simulink model "darko_test_integrateur"  (R2021b)
settings: Solver=VariableStepAuto  StartTime=0.0  StopTime=30  RelTol=1e-3
values from neighbouring files (symbols this model uses):
  drone = generateDarko()    [main_linearisation.m]
  initial_state = [p_initial; v_initial; q_initial; omega_initial]    [main_linearisation.m]
  K_complet = [K(:,1:6), zeros(4,1), K(:,7:12)]    [main_linearisation.m]
  S_complet = [S(1:6,1:6), zeros(6,1), S(1:6,7:12); zeros(1,13); S(7:12,1:6), zeros(6,1), S(7:12,7:12)]    [main_linearisation.m]
  u_eq = drone.G*drone.MASS/(2*drone.Fb(1,1)) * [1;1;0;0]    [main_linearisation.m]
  x_eq = [[0; 0; 0]; [0; 0; 0]; eul2quat([yaw, pitch, roll])'; [0; 0; 0]]    [main_linearisation.m]
libraries: simulink_extras x3, sharedtransform x1
settings Model: Creator=florian  LastModifiedBy=florian
settings SolverCC: AlgebraicLoopSolver=TrustRegion
settings DebuggingCC: SFMachineParentedDataDiag=warning

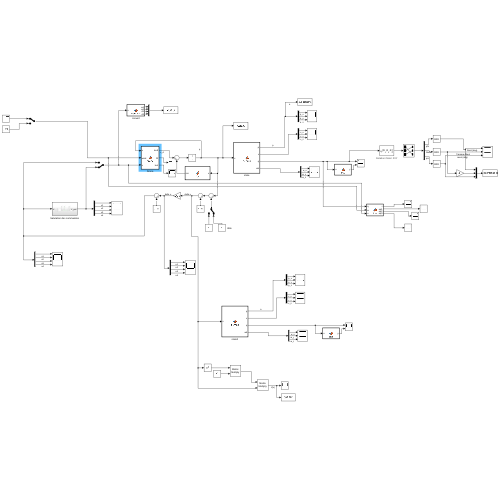
[thumbnail: Simulink's stored preview of the top-level diagram]
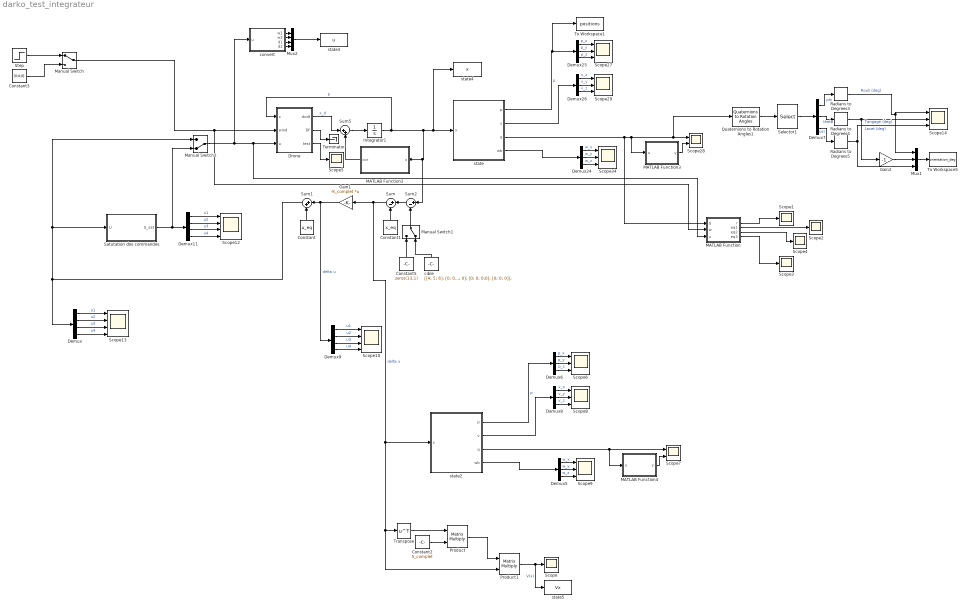
== system darko_test_integrateur ==
  Constant : Constant  Value=u_eq
  Constant1 : Constant  Value=x_eq
  Constant2 : Constant  Value=S_complet
  Constant3 : Constant  Value=[0;0;0]
  Constant5 : Constant  Value=zeros(13,1)
  Demux : Demux
  Demux11 : Demux
  Demux{5..8,24..26} (7 alike) : Demux  Outputs=3
  Demux9 : Demux
  Drone : MATLAB Function  TreatAsAtomicUnit=on
  Gain1 : Gain  Gain=-K_complet  Multiplication=Matrix(K*u) (u vector)
  Gain2 : Gain  Gain=-1
  Integrator1 : Integrator  InitialCondition=initial_state
  MATLAB Function : MATLAB Function  TreatAsAtomicUnit=on
  MATLAB Function2 : MATLAB Function  TreatAsAtomicUnit=on
  MATLAB Function3 : MATLAB Function  TreatAsAtomicUnit=on
  MATLAB Function4 : MATLAB Function  TreatAsAtomicUnit=on
  Manual Switch : ManualSwitch
  Manual Switch1 : ManualSwitch  CurrentSetting=0
  Manual Switch2 : ManualSwitch  CurrentSetting=0
  Mux1 : Mux  Inputs=3
  Mux2 : Mux
  Product : Product  Multiplication=Matrix(*)
  Product1 : Product  Multiplication=Matrix(*)
  Quaternions to Rotation Angles1 : sharedtransform/Quaternions to Rotation Angles  rotationOrder=ZXY  aMode=aMode
      settings: SourceProductBaseCode=AE,PW,DR,MT,UV,VE
  Radians to Degrees3 : simulink_extras/Transformations/Radians to Degrees
  Radians to Degrees4 : simulink_extras/Transformations/Radians to Degrees
  Radians to Degrees5 : simulink_extras/Transformations/Radians to Degrees
  Satutation des commandes : Subsystem
  Scope{,1..5} (6 alike) : Scope
  Scope10 : Scope  NumInputPorts=4
  Scope12 : Scope  NumInputPorts=4
  Scope13 : Scope  NumInputPorts=4
  Scope{6,8..9,14,27,29,34} (7 alike) : Scope  NumInputPorts=3
  Scope28 : Scope  NumInputPorts=2
  Scope7 : Scope  NumInputPorts=2
  Selector1 : Selector  InputPortWidth=3  IndexOptions=Index vector (dialog)  Indices=[2 3 1]  OutputSizes=1
  Step : Step  Time=10  Before=[0;0;0]  After=[0;0;-10]  SampleTime=0
  Sum : Sum  Inputs=|+-
  Sum1 : Sum  Inputs=|++
  Sum2 : Sum  Inputs=|+-
  Sum5 : Sum  Inputs=|++
  Terminator : Terminator
  To Workspace1 : ToWorkspace  VariableName=positions  SampleTime=-1
  To Workspace5 : ToWorkspace  VariableName=orientation_deg  SampleTime=-1
  Transpose : Math  Operator=transpose  SaturateOnIntegerOverflow=on
  cible : Constant  Value=[[4; 5; 6]; [0; 0; 0]; [0; 0; 0;0]; [0; 0; 0]];
  convert : MATLAB Function  TreatAsAtomicUnit=on
  state : MATLAB Function  TreatAsAtomicUnit=on
  state2 : MATLAB Function  TreatAsAtomicUnit=on
  state3 : ToWorkspace  VariableName=u  SampleTime=-1
  state4 : ToWorkspace  VariableName=x  SampleTime=-1
  state5 : ToWorkspace  VariableName=Vx  SampleTime=-1
  wires:
  Sum5/1 -> Integrator1/1
  MATLAB Function2/1(cor) -> Sum5/2
  Drone/1(dxdt) -> Sum5/1  "x_d"
  Integrator1/1 -> Drone/1(x), state4/1, state/1(x), Sum2/1, MATLAB Function2/1(x)  "p"
  Demux25/3 -> Scope27/3  "p_z"
  Demux26/2 -> Scope29/2  "v_y"
  Demux24/1 -> Scope34/1  "w_x"
  MATLAB Function3/1(y) -> Scope28/2
  state/3(q) -> MATLAB Function/1(q), MATLAB Function3/1(u), Quaternions to Rotation Angles1/1, Scope28/1
  Demux25/1 -> Scope27/1  "p_x"
  state/4(wb) -> Demux24/1
  Demux24/2 -> Scope34/2  "w_y"
  Demux24/3 -> Scope34/3  "w_z"
  state/2(v) -> Demux26/1
  Demux25/2 -> Scope27/2  "p_y"
  Demux26/3 -> Scope29/3  "v_z"
  Demux26/1 -> Scope29/1  "v_x"
  Gain1/1 -> Demux9/1, Sum1/1  "delta u"
  Constant/1 -> Sum1/2
  Constant1/1 -> Sum/2
  Demux6/3 -> Scope6/3  "p_z"
  Demux8/2 -> Scope8/2  "v_y"
  state2/3(q) -> MATLAB Function4/1(u), Scope7/1
  state2/4(wb) -> Demux5/1
  MATLAB Function4/1(y) -> Scope7/2
  Demux5/2 -> Scope9/2  "w_y"
  Demux8/3 -> Scope8/3  "v_z"
  Demux6/1 -> Scope6/1  "p_x"
  Demux5/1 -> Scope9/1  "w_x"
  Demux8/1 -> Scope8/1  "v_x"
  state2/1(p) -> Demux6/1  "p"
  Demux6/2 -> Scope6/2  "p_y"
  Demux5/3 -> Scope9/3  "w_z"
  state2/2(v) -> Demux8/1
  Demux9/3 -> Scope10/3  "u3"
  Demux9/4 -> Scope10/4  "u4"
  Demux9/1 -> Scope10/1  "u1"
  Demux9/2 -> Scope10/2  "u2"
  Product1/1 -> state5/1, Scope/1  "V(x)"
  Transpose/1 -> Product/1
  Constant2/1 -> Product/2
  Product/1 -> Product1/1
  Manual Switch/1 -> MATLAB Function/2(w), Drone/2(wind)
  Step/1 -> Manual Switch/1
  Constant3/1 -> Manual Switch/2
  cible/1 -> Manual Switch1/2
  Manual Switch1/1 -> Sum2/2
  Constant5/1 -> Manual Switch1/1
  Sum2/1 -> Sum/1
  Demux/1 -> Scope13/1  "u1"
  Demux11/2 -> Scope12/2  "u2"
  Demux11/4 -> Scope12/4  "u4"
  Demux/2 -> Scope13/2  "u2"
  Demux/4 -> Scope13/4  "u4"
  Demux11/1 -> Scope12/1  "u1"
  Demux/3 -> Scope13/3  "u3"
  Sum1/1 -> Satutation des commandes/1(U), Manual Switch2/1, Demux/1
  Satutation des commandes/1(U_sat) -> Manual Switch2/2, Demux11/1
  Demux11/3 -> Scope12/3  "u3"
  Manual Switch2/1 -> convert/1(u), MATLAB Function/3(u), Drone/3(u)
  Sum/1 -> Product1/2, Transpose/1, state2/1(x), Gain1/1  "delta x"
  Demux7/2 -> Radians to Degrees4/1  "theta"
  Radians to Degrees4/1 -> Gain2/1, Scope14/2  "Tangage (deg)"
  Gain2/1 -> Mux1/2
  Mux1/1 -> To Workspace5/1
  Radians to Degrees5/1 -> Mux1/3, Scope14/3  "Lacet (deg)"
  Quaternions to Rotation Angles1/1 -> Selector1/1
  Demux7/3 -> Radians to Degrees5/1  "psi"
  Selector1/1 -> Demux7/1
  Demux7/1 -> Radians to Degrees3/1  "phi"
  Radians to Degrees3/1 -> Mux1/1, Scope14/1  "Rouli (deg)"
  state/1(p) -> To Workspace1/1, Demux25/1  "p"
  convert/2(w2) -> Mux2/2
  convert/4(d2) -> Mux2/4
  convert/3(d1) -> Mux2/3
  Mux2/1 -> state3/1
  convert/1(w1) -> Mux2/1
  MATLAB Function/1(r) -> Scope1/1
  MATLAB Function/2(eq1) -> Scope2/1
  MATLAB Function/4(eq3) -> Scope3/1
  MATLAB Function/3(eq2) -> Scope4/1
  Drone/2(Df) -> Terminator/1
  Drone/3(test) -> Scope5/1

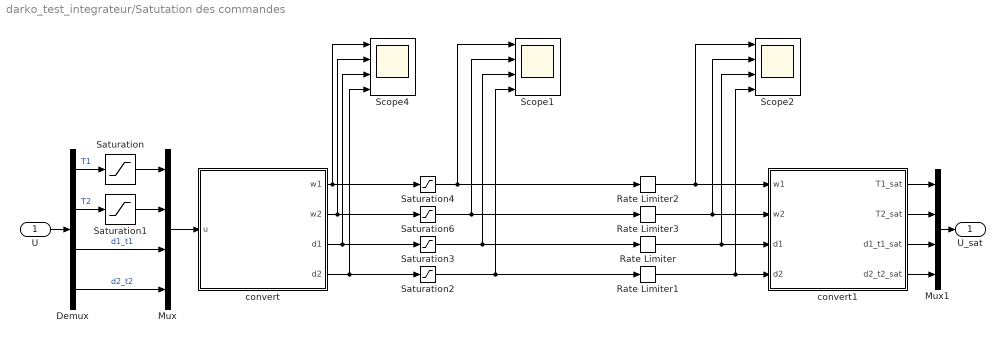
== system darko_test_integrateur/Satutation des commandes ==
  U : Inport
  Demux : Demux
  Mux : Mux
  Mux1 : Mux
  Rate Limiter : RateLimiter  RisingSlewLimit=drone.ELEVON_RATE_CHANGE  FallingSlewLimit=-drone.ELEVON_RATE_CHANGE  SampleTimeMode=inherited
  Rate Limiter1 : RateLimiter  RisingSlewLimit=drone.ELEVON_RATE_CHANGE  FallingSlewLimit=-drone.ELEVON_RATE_CHANGE  SampleTimeMode=inherited
  Rate Limiter2 : RateLimiter  RisingSlewLimit=drone.MOTOR_RATE_CHANGE  FallingSlewLimit=-drone.MOTOR_RATE_CHANGE  SampleTimeMode=inherited
  Rate Limiter3 : RateLimiter  RisingSlewLimit=drone.MOTOR_RATE_CHANGE  FallingSlewLimit=-drone.MOTOR_RATE_CHANGE  SampleTimeMode=inherited
  Saturation : Saturate  UpperLimit=100  LowerLimit=0.001
  Saturation1 : Saturate  UpperLimit=100  LowerLimit=0.001
  Saturation2 : Saturate  UpperLimit=30*(pi/180)  LowerLimit=-30*(pi/180)
  Saturation3 : Saturate  UpperLimit=30*(pi/180)  LowerLimit=-30*(pi/180)
  Saturation4 : Saturate  UpperLimit=1000  LowerLimit=200
  Saturation6 : Saturate  UpperLimit=1000  LowerLimit=200
  Scope1 : Scope  NumInputPorts=4
  Scope2 : Scope  NumInputPorts=4
  Scope4 : Scope  NumInputPorts=4
  convert : MATLAB Function  TreatAsAtomicUnit=on
  convert1 : MATLAB Function  TreatAsAtomicUnit=on
  U_sat : Outport
  wires:
  U/1 -> Demux/1
  Demux/4 -> Mux/4  "d2_t2"
  Demux/1 -> Saturation/1  "T1"
  Demux/3 -> Mux/3  "d1_t1"
  Demux/2 -> Saturation1/1  "T2"
  Saturation/1 -> Mux/1
  Mux/1 -> convert/1(u)
  convert/1(w1) -> Saturation4/1, Scope4/1
  Saturation3/1 -> Rate Limiter/1, Scope1/3
  convert/2(w2) -> Scope4/2, Saturation6/1
  convert/3(d1) -> Scope4/3, Saturation3/1
  convert/4(d2) -> Saturation2/1, Scope4/4
  convert1/1(T1_sat) -> Mux1/1
  convert1/4(d2_t2_sat) -> Mux1/4
  Mux1/1 -> U_sat/1
  Saturation1/1 -> Mux/2
  convert1/2(T2_sat) -> Mux1/2
  convert1/3(d1_t1_sat) -> Mux1/3
  Saturation2/1 -> Rate Limiter1/1, Scope1/4
  Rate Limiter/1 -> Scope2/3, convert1/3(d1)
  Saturation6/1 -> Rate Limiter3/1, Scope1/2
  Saturation4/1 -> Rate Limiter2/1, Scope1/1
  Rate Limiter1/1 -> Scope2/4, convert1/4(d2)
  Rate Limiter2/1 -> Scope2/1, convert1/1(w1)
  Rate Limiter3/1 -> Scope2/2, convert1/2(w2)

== matlab function darko_test_integrateur/state ==
  data: x input; p output; v output; q output; wb output
function [p, v, q, wb] = demux(x)
%#codegen

p = x(1:3);
v = x(4:6);
q  = x(7:10);
wb = x(11:13);

== matlab function darko_test_integrateur/MATLAB Function ==
  data: q input; w input; u input; r output; drone parameter; eq1 output; eq2 output; eq3 output
function [r,eq1,eq2,eq3] = fcn(q,w,u,drone)
%#codegen
theta=2*asin(q(3));

rho = drone.RHO;
Swet   = drone.WET_SURFACE;
Sp = pi*drone.PROP_RADIUS^2;
Thetam = drone.ELEVON_MEFFICIENCY;
Thetaf = drone.ELEVON_FEFFICIENCY;
Cd0 = drone.PHI(1,1);
Cl0 = drone.PHI(3,3);
g = drone.G;
% vehicle mass
m = drone.MASS;


mu=(1-Thetaf(2)/Thetam(2))*(Swet*Cl0*rho)/(2*m*g);

r=mu*w(1)*sin(theta)-(mu*w(3)-1)*cos(theta);

wx_b = cos(theta)*w(1) + sin(theta)*w(3);
wz_b = cos(theta)*w(3) - sin(theta)*w(1);

eq1=rho*Thetam(2)*(u(3)/u(1))*wx_b + rho*wz_b + (1/Sp)*Thetam(2)*u(3);

eq2 = sin(theta)*m*g +2*(1-(Swet/4*Sp)*Cd0)*u(1) + (1/2)*rho*Swet*Cd0*(wx_b-Thetaf(2)*(u(1)/u(3))*wz_b);

eq3 = -cos(theta)*m*g +2*(-(Swet/4*Sp)*Cl0*Thetaf(2))*u(3) + (1/2)*rho*Swet*Cl0*(wz_b + Thetaf(2)*(u(1)/u(3))*wx_b);

== matlab function darko_test_integrateur/Drone ==
  data: x input; wind input; u input; dxdt output; drone parameter; Df output; test output
function [dxdt, Df, test]   = drone(x,wind, u, drone)

%% physical constants
% gravity
g = drone.G;
% vehicle mass
m = drone.MASS;
% vehicle inertia matrix
J = drone.INERTIA; % [3x3 real symmetric] in body axis

rho = drone.RHO;
Swet   = drone.WET_SURFACE;
Sp = pi*drone.PROP_RADIUS^2;
Thetam = drone.ELEVON_MEFFICIENCY;
Thetaf = drone.ELEVON_FEFFICIENCY;
Cd0 = drone.PHI(1,1);
Cl0 = drone.PHI(3,3);
dR = drone.CENTRAGE ;

af = drone.Fb(1,1);
bf = drone.Fb(3,3);

%% state demultiplexing
% p = x(1:3);
v = x(4:6);
q  = x(7:10);
wb = x(11:13);

Rq = q2dcm(q);

[Fp, Mp] = external_force_moment(x, u, wind, drone);

% position
dpdt = v;

Df = -(1/4)*rho*Swet*[-2*Cd0 0 Cd0*Thetaf(2)*((u(3)/u(1))+(u(4)/u(2))); 0 0 0; -Thetaf(2)*Cl0*((u(3)/u(1))+(u(4)/u(2))) 0 -2*Cl0];
test=norm(Rq*Df*Rq'*norm(wind)*wind)
% kinematics
dvdt =  -[0;0;g] + (1/m)*Rq*drone.Fb*u + (1/m)*Rq*Df*Rq'*norm(wind)*wind; 

%% quaternion derivative
eta = q(1);
eps = q(2:4);

dqdt = (1/2)*[-eps'; eta*eye(3) + skew_sym(eps)]*wb;

%% angular velocity derivative
Dm = -(1/4)*rho*Swet*[0 0 0; dR*Thetam(2)*Cl0*((u(3)/u(1))+(u(4)/u(2))) 0 -2*dR*Cl0; 0 0 0];
% kinematics
dwdt = inv(J)*(-cross(wb, J*wb) + (drone.Mb*u) + Dm*Rq'*norm(wind)*wind);


%% derivative multiplexing
dxdt = [dpdt; dvdt; dqdt; dwdt] ;

== matlab function darko_test_integrateur/MATLAB Function4 ==
  data: u input; y output
function y = fcn(u)
%#codegen

y = norm(u);

== matlab function darko_test_integrateur/state2 ==
  data: x input; p output; v output; q output; wb output
function [p, v, q, wb] = demux(x)
%#codegen

p = x(1:3);
v = x(4:6);
q  = x(7:10);
wb = x(11:13);

== matlab function darko_test_integrateur/Satutation des commandes/convert ==
  data: u input; w1 output; drone parameter; w2 output; d1 output; d2 output
function [w1, w2, d1, d2] = convert(u, drone)
%#codegen
kf = drone.PROP_KP;

T1 = u(1);
T2 = u(2);
d1_T1 = u(3);
d2_T2 = u(4);

w1 = sqrt(T1/kf);
w2 = sqrt(T2/kf);
d1 = d1_T1/T1;
d2 = d2_T2/T2;

== matlab function darko_test_integrateur/Satutation des commandes/convert1 ==
  data: w1 input; w2 input; d1 input; d2 input; T1_sat output; T2_sat output; drone parameter; d1_t1_sat output; d2_t2_sat output
function [T1_sat, T2_sat, d1_t1_sat, d2_t2_sat] = convert2(w1, w2, d1, d2, drone)
%#codegen
kf = drone.PROP_KP;

T1_sat = kf*w1^2;
d1_t1_sat = d1*T1_sat;
T2_sat = kf*w2^2;
d2_t2_sat = d2*T2_sat;

== matlab function darko_test_integrateur/MATLAB Function2 ==
  data: x input; cor output
function cor  = fcn(x)
%#codegen
q  = x(7:10);
n = norm(q);
mismatch = 1-n;
cor = [0;0;0; 0;0;0; mismatch*q; 0;0;0];

== matlab function darko_test_integrateur/MATLAB Function3 ==
  data: u input; y output
function y = fcn(u)
%#codegen

y = norm(u);

== matlab function darko_test_integrateur/convert ==
  data: u input; w1 output; drone parameter; w2 output; d1 output; d2 output
function [w1, w2, d1, d2] = convert(u, drone)
%#codegen
kf = drone.PROP_KP;

T1 = max(u(1),0);
T2 = max(u(2),0);
d1_T1 = u(3);
d2_T2 = u(4);

w1 = sqrt(T1/kf)*60/(2*pi);
w2 = sqrt(T2/kf)*60/(2*pi);
d1 = d1_T1/T1 *(360/(2*pi));
d2 = d2_T2/T2*(360/(2*pi));
